simulink model "foc_sensorless_am13x"  (R2025b)
settings: Solver=FixedStepAuto  StartTime=0.0  StopTime=10  RelTol=1e-3  EnableMultiTasking=on
PostLoadFcn:
  | foc_sensorless_am13x_data;
values from neighbouring files (symbols this model uses):
  inverter = mcb.getInverterParameters('BoostXL-DRV8305')    [foc_sensorless_am13x_data.m]
  PI_params = mcb.getPIControllerParameters(pmsm, inverter, PU_System, T_pwm, Ts, Ts_speed)    [foc_sensorless_am13x_data.m]
  pmsm = mcb.getPMSMParameters('Teknic2310P')    [foc_sensorless_am13x_data.m]
  PU_System = mcb.getPUSystemParameters(pmsm, inverter)    [foc_sensorless_am13x_data.m]
  RAMP_STEP_SIZE = Id_init_assumed / N_ramp_steps    (= 0.00025)    [foc_sensorless_am13x_data.m]
  Speed_openLoop_RPM = Speed_openLoop_PU*pmsm.N_base    [foc_sensorless_am13x_data.m]
  T_pwm = 1 / PWM_frequency    (= 5e-05)    [foc_sensorless_am13x_data.m]
  Tclosedloop_stepTime = 5    [foc_sensorless_am13x_data.m]
  Ts = T_pwm    (= 5e-05)    [foc_sensorless_am13x_data.m]
  Ts_motor = T_pwm / 2    (= 2.5e-05)    [foc_sensorless_am13x_data.m]
  Ts_speed = 10 * Ts    (= 0.0005)    [foc_sensorless_am13x_data.m]
  Tspeedchange_stepTime = 7    [foc_sensorless_am13x_data.m]
undefined symbols (not defined in the file or in its folder): ADC_0_INST, DL_ADC_clearInterruptStatus, DL_ADC_INT_NUMBER1, DL_MCPWM_disableTBCLK, target
libraries: mcbcontrolslib x11, mcbeeMathTransformLib x5, simulink x5, slpidlib x3, peripheral_library_blocks_am13x x2, mcbhdlcontrolslib x2, mcbsensorlessestimatorlib x2, mcbpositiondecoderlib x2, mcbplantlib x1, autolibpmsmexterior x1, simulink_extras x1
(part 2 of 2)

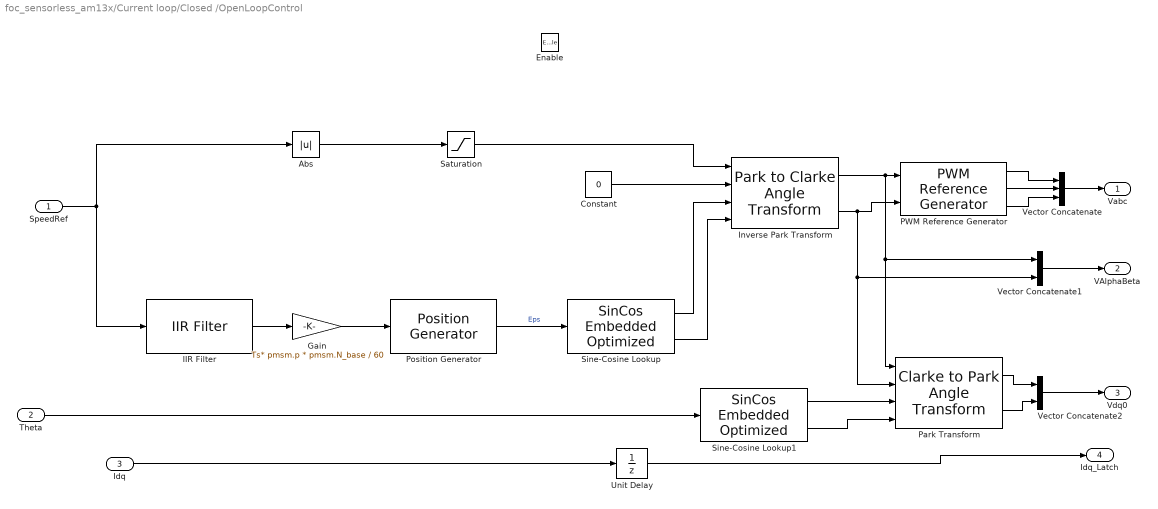
== system foc_sensorless_am13x/Current loop/Closed /OpenLoopControl ==
  SpeedRef : Inport
  Theta : Inport  Port=2
  Idq : Inport  Port=3
  Enable : EnablePort  StatesWhenEnabling=reset
  Abs : Abs  SaturateOnIntegerOverflow=off
  Constant : Constant  Value=0  OutDataTypeStr=dataType
  Gain : Gain  Gain=Ts* pmsm.p * pmsm.N_base / 60  RndMeth=Simplest  OutDataTypeStr=Inherit: Same as input
  IIR Filter : mcbhdlcontrolslib/IIR Filter  VariantControl=Low Pass Filter  VariantSelect=Low-pass  FilterConstantInputType=Specify via dialog  Filter_constant=0.01  advancedSettings=off  Ts=50e-6  cutOff_freq=32.1525
  Inverse Park Transform : mcbeeMathTransformLib/Park to Clarke Angle Transform  AxisAlignment=D-axis  UseWithEmbedded=on  PhaseInput=Two inputs  ThetaInput=Sine and Cosine electrical position  AngleInput=Per-unit  N_points=1024
      settings: LibrarySourceBlock=mcbhdllib/Controls/Math Transforms/Inverse Park Transform
  PWM Reference Generator : mcbcontrolslib/PWM Reference Generator  inSignal=Valphabeta  modType=SVM: space vector modulation
      settings: LibrarySourceBlock=mcblib/Controls/Math Transforms/PWM Reference Generator
  Park Transform : mcbeeMathTransformLib/Clarke to Park Angle Transform  AxisAlignment=D-axis  UseWithEmbedded=on  PhaseInput=Two inputs  ThetaInput=Sine and Cosine electrical position  AngleInput=Per-unit  N_points=1024
      settings: LibrarySourceBlock=mcbhdllib/Controls/Math Transforms/Park Transform
  Position Generator : mcbhdlcontrolslib/Position Generator  AngleOutput=Per-unit  ExternalReset=none  Offset=0
  Saturation : Saturate  LowerLimit=pmsm.V_boost  RndMeth=Simplest
  Sine-Cosine Lookup : mcbcontrolslib/SinCos Embedded Optimized  LabelModeActiveChoice=MCB_Sin  OptforProc=off  ApproximationMethod=None  UserApproxMethod=Lookup  ApproxStatus=None  InterpMethod=Linear point-slope  NumberOfDataPoints=16  NumberOfIterations=11  RemoveProtectionAgainstOutOfRangeInput=off  TableDataTypeStr=Inherit: Inherit via input  AngleInput=Per-unit  ThetaDataType=single  N_points=1024  DatatypeInput=Inherit from input  Datatype=Inherit: Same as input
      settings: LibrarySourceBlock=mcblib/Controls/Math Transforms/Sine-Cosine Lookup
  Sine-Cosine Lookup1 : mcbcontrolslib/SinCos Embedded Optimized  LabelModeActiveChoice=MCB_Sin  OptforProc=off  ApproximationMethod=None  UserApproxMethod=Lookup  ApproxStatus=None  InterpMethod=Linear point-slope  NumberOfDataPoints=16  NumberOfIterations=11  RemoveProtectionAgainstOutOfRangeInput=off  TableDataTypeStr=Inherit: Inherit via input  AngleInput=Per-unit  ThetaDataType=single  N_points=1024  DatatypeInput=Inherit from input  Datatype=Inherit: Same as input
      settings: LibrarySourceBlock=mcblib/Controls/Math Transforms/Sine-Cosine Lookup
  Unit Delay : UnitDelay  SampleTime=-1  HasFrameUpgradeWarning=on
  Vector Concatenate : Concatenate  NumInputs=3
  Vector Concatenate1 : Concatenate
  Vector Concatenate2 : Concatenate
  Vabc : Outport
  VAlphaBeta : Outport  Port=2
  Vdq0 : Outport  Port=3
  Idq_Latch : Outport  Port=4
  wires:
  SpeedRef/1 -> IIR Filter/1, Abs/1
  Abs/1 -> Saturation/1
  Constant/1 -> Inverse Park Transform/2
  IIR Filter/1 -> Gain/1
  Gain/1 -> Position Generator/1
  Position Generator/1 -> Sine-Cosine Lookup/1  "Eps"
  Sine-Cosine Lookup/1 -> Inverse Park Transform/3
  Sine-Cosine Lookup/2 -> Inverse Park Transform/4
  Inverse Park Transform/1 -> Park Transform/1, Vector Concatenate1/1, PWM Reference Generator/1
  Inverse Park Transform/2 -> Park Transform/2, Vector Concatenate1/2, PWM Reference Generator/2
  PWM Reference Generator/3 -> Vector Concatenate/3
  PWM Reference Generator/2 -> Vector Concatenate/2
  PWM Reference Generator/1 -> Vector Concatenate/1
  Vector Concatenate/1 -> Vabc/1
  Vector Concatenate1/1 -> VAlphaBeta/1
  Park Transform/1 -> Vector Concatenate2/1
  Park Transform/2 -> Vector Concatenate2/2
  Vector Concatenate2/1 -> Vdq0/1
  Sine-Cosine Lookup1/1 -> Park Transform/3
  Sine-Cosine Lookup1/2 -> Park Transform/4
  Theta/1 -> Sine-Cosine Lookup1/1
  Saturation/1 -> Inverse Park Transform/1
  Idq/1 -> Unit Delay/1
  Unit Delay/1 -> Idq_Latch/1

== system foc_sensorless_am13x/Current loop/Closed /OutputScaling ==
  VabcClosed : Inport
  VabcOpen : Inport  Port=2
  EnCl : Inport  Port=3  OutDataTypeStr=boolean
  Mode : Inport  Port=4
  Add2 : Sum
  Constant : Constant  Value=0.5  OutDataTypeStr=dataType
  Current Offset Calib : Constant  Value=[0.5 0.5 0.5]  OutDataTypeStr=dataType
  Gain : Gain  Gain=0.5  RndMeth=Simplest  OutDataTypeStr=Inherit: Same as input
  Switch : Switch  Criteria=u2 > Threshold  SaturateOnIntegerOverflow=off  InputSameDT=off
  Switch3 : Switch  Criteria=u2 > Threshold  SaturateOnIntegerOverflow=off  InputSameDT=off
  Vabc_PU : Outport  OutDataTypeStr=single  VectorParamsAs1DForOutWhenUnconnected=off
  wires:
  VabcClosed/1 -> Switch/1
  EnCl/1 -> Switch/2
  Gain/1 -> Add2/1
  VabcOpen/1 -> Switch/3
  Constant/1 -> Add2/2
  Switch/1 -> Gain/1
  Switch3/1 -> Vabc_PU/1
  Mode/1 -> Switch3/2
  Add2/1 -> Switch3/1
  Current Offset Calib/1 -> Switch3/3

== system foc_sensorless_am13x/Current loop/Closed /Sensorless algorithms to calculate position and speed ==
  note: Try different sensorless algorithms
  EnPWM : Inport
  VI_fb : Inport  Port=2
  Data Store Memory : DataStoreMemory  DataStoreName=Enable  WriteAfterWriteMsg=warning  ShowAdditionalParam=off
  Data Store Write : DataStoreWrite  DataStoreName=Enable  DataStoreElements=Enable  IndexOptions=Index vector (dialog)  Indices=1  OutputSizes=1
  Demux : Demux  Outputs=2
  EstimatorSelector : Constant  Value=2  OutDataTypeStr=uint32
  Extended EMF Observer : Subsystem
  Flux Observer : Subsystem
  Merge : Merge  Inputs=3
  Sliding Mode Observer : Subsystem
  Switch Case : SwitchCase  CaseConditions={0,1,2}  ShowDefaultCase=off
  Pos_PU : Outport
  speed_PU : Outport  Port=2
  wires:
  Switch Case/3 -> Extended EMF Observer/Action
  Extended EMF Observer/1(Position/Speed) -> Merge/3
  VI_fb/1 -> Sliding Mode Observer/1(InputSignals), Flux Observer/1(InputSignals), Extended EMF Observer/1(InputSignals)
  Switch Case/1 -> Sliding Mode Observer/Action
  Switch Case/2 -> Flux Observer/Action
  Merge/1 -> Demux/1
  Flux Observer/1(Position/Speed) -> Merge/2
  Sliding Mode Observer/1(Position/Speed) -> Merge/1
  EstimatorSelector/1 -> Switch Case/1
  Demux/2 -> speed_PU/1
  Demux/1 -> Pos_PU/1
  EnPWM/1 -> Data Store Write/1

== system foc_sensorless_am13x/Current loop/Create Buffer/Data ==
  Data : Inport
  Data_width : Inport  Port=2
  Action Port : ActionPort  ActionPortLabel=else
  Mux : Mux  Inputs=2
  Start : Constant  Value=hex2dec('0000')  OutDataTypeStr=uint16
  Data_out : Outport  VectorParamsAs1DForOutWhenUnconnected=off
  Iteration : Outport  Port=2  VectorParamsAs1DForOutWhenUnconnected=off
  wires:
  Start/1 -> Mux/2
  Mux/1 -> Data_out/1
  Data/1 -> Mux/1
  Data_width/1 -> Iteration/1

== system foc_sensorless_am13x/Current loop/Create Buffer/Data_Conditioning ==
  In1 : Inport
  Data Type Conversion : DataTypeConversion  OutDataTypeStr=fixdt(1,32,12)  RndMeth=Simplest  SaturateOnIntegerOverflow=off
  Data Type Conversion3 : DataTypeConversion  OutDataTypeStr=uint16  ConvertRealWorld=Stored Integer (SI)  RndMeth=Simplest  SaturateOnIntegerOverflow=off
  Out1 : Outport  VectorParamsAs1DForOutWhenUnconnected=off
  wires:
  In1/1 -> Data Type Conversion/1
  Data Type Conversion3/1 -> Out1/1
  Data Type Conversion/1 -> Data Type Conversion3/1

== system foc_sensorless_am13x/Current loop/Create Buffer/End ==
  Data : Inport
  Data_width : Inport  Port=2
  Action Port : ActionPort  ActionPortLabel=elseif(u1 == 599)
  Bias : Bias  Bias=1  SaturateOnIntegerOverflow=off
  Mux : Mux  Inputs=2
  Start : Constant  Value=hex2dec('4545')  OutDataTypeStr=uint16
  Data_out : Outport  VectorParamsAs1DForOutWhenUnconnected=off
  Iteration : Outport  Port=2  VectorParamsAs1DForOutWhenUnconnected=off
  wires:
  Mux/1 -> Data_out/1
  Data_width/1 -> Bias/1
  Start/1 -> Mux/2
  Bias/1 -> Iteration/1
  Data/1 -> Mux/1

== system foc_sensorless_am13x/Current loop/Create Buffer/Start ==
  Data : Inport
  Data_width : Inport  Port=2
  Action Port : ActionPort  ActionPortLabel=if(u1 == 0)
  Bias : Bias  Bias=1  SaturateOnIntegerOverflow=off
  End : Constant  Value=hex2dec('5353')  OutDataTypeStr=uint16
  Mux : Mux  Inputs=2
  Data_out : Outport  VectorParamsAs1DForOutWhenUnconnected=off
  Iteration : Outport  Port=2  VectorParamsAs1DForOutWhenUnconnected=off
  wires:
  End/1 -> Mux/1
  Mux/1 -> Data_out/1
  Data_width/1 -> Bias/1
  Bias/1 -> Iteration/1
  Data/1 -> Mux/2

== system foc_sensorless_am13x/Current loop/Serial Send/While Iterator Subsystem ==
  note: UART configuration is done via HAL APIs
      | - Its hardcoded for 5e6 baud refer the source am13x_serial_util.c
  Data : Inport
  Iteration : Inport  Port=2
  Add : Sum  Inputs=+-  OutDataTypeStr=Inherit: Same as first input
  HAL Serial API Caller : CFunction  CodeGenUsesSimCustomCode=off  CodegenOutputCode=mw_am13x_serial_Send((const uint8_t *)&serialIn, sizeof(uint16_t));  CustomHeaderFile=|  CustomSourceFile=am13x_serial_util.c
      | dl_mcpwm.h
      | hw_memmap.h
      | ti_sdk_dl_config.h
      | Uart_Hal.h
      | dl_gpio.h
      | mw_am13x_serial.h
  Index Vector : MultiPortSwitch  Inputs=1  SaturateOnIntegerOverflow=off  InputSameDT=off
  While Iterator : WhileIterator  MaxIters=-1  WhileBlockType=do-while  ShowIterationPort=on  OutputDataType=int16
  wires:
  While Iterator/1 -> Add/2, Index Vector/1
  Data/1 -> Index Vector/2
  Add/1 -> While Iterator/1
  Iteration/1 -> Add/1
  Index Vector/1 -> HAL Serial API Caller/1

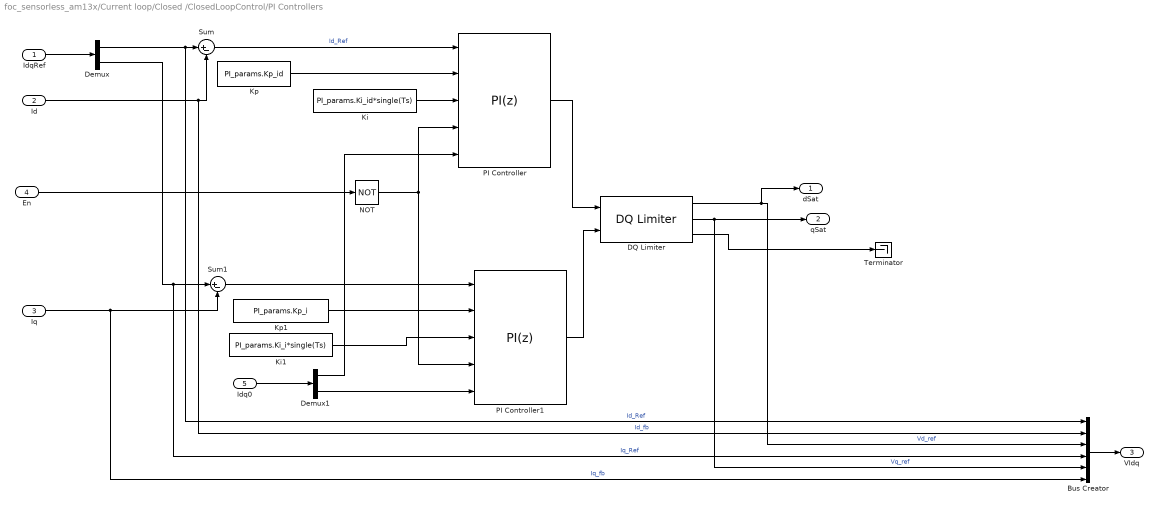
== system foc_sensorless_am13x/Current loop/Closed /ClosedLoopControl/PI Controllers ==
  IdqRef : Inport
  Id : Inport  Port=2
  Iq : Inport  Port=3
  En : Inport  Port=4
  Idq0 : Inport  Port=5
  Bus Creator : BusCreator  Inputs=6
  DQ Limiter : mcbcontrolslib/DQ Limiter  satMethodInputType=Specify via dialog  satMethodSelected=D-Q equivalence  satLimitInputType=Specify via dialog  Vmax=.95
      settings: LibrarySourceBlock=mcblib/Controls/Control Reference/DQ Limiter
  Demux : Demux  Outputs=2
  Demux1 : Demux  Outputs=2
  Ki : Constant  Value=PI_params.Ki_id*single(Ts)  OutDataTypeStr=dataType  SampleTime=-1
  Ki1 : Constant  Value=PI_params.Ki_i*single(Ts)  OutDataTypeStr=dataType  SampleTime=-1
  Kp : Constant  Value=PI_params.Kp_id  OutDataTypeStr=dataType  SampleTime=-1
  Kp1 : Constant  Value=PI_params.Kp_i  OutDataTypeStr=dataType  SampleTime=-1
  NOT : Logic  Operator=NOT  IconShape=distinctive  AllPortsSameDT=off  OutDataTypeStr=boolean
  PI Controller : slpidlib/PID Controller  Controller=PI  Form=Parallel  TimeDomain=Discrete-time  UseExternalTs=off  SampleTime=-1  IntegratorMethod=Forward Euler  FilterMethod=Forward Euler  ControllerParametersSource=external  P=1  I=1  UseKiTs=on  D=0  UseExternalDerivativeSource=off  N=100  UseFilter=on  TunerSelectOption=Transfer Function Based (PID Tuner App)  InitialConditionSource=external  InitialConditionForIntegrator=0  InitialConditionForFilter=0  DifferentiatorICPrevScaledInput=0  ExternalReset=level  TrackingMode=off  Kt=1  LimitOutput=on  SatLimitsSource=internal  UpperSaturationLimit=1  LowerSaturationLimit=-1  LinearizeAsGain=on  AntiWindupMode=clamping  Kb=1  LimitIntegrator=off  UpperIntegratorSaturationLimit=inf  LowerIntegratorSaturationLimit=-inf  RndMeth=Simplest  POutMin=[]  POutMax=[]  IOutMin=[]  IOutMax=[]  DOutMin=[]  DOutMax=[]  NOutMin=[]  NOutMax=[]  SumOutMin=[]  SumOutMax=[]  SaturationOutDataTypeStr=Inherit: Inherit via back propagation  SaturationOutMin=[]  SaturationOutMax=[]  PParamMin=[]  PParamMax=[]  IParamMin=[]  IParamMax=[]  DParamMin=[]  DParamMax=[]  NParamMin=[]  NParamMax=[]  KbParamMin=[]  KbParamMax=[]  KtParamMin=[]  KtParamMax=[]  KbOutMin=[]  KbOutMax=[]  KtOutMin=[]  KtOutMax=[]  IntegratorOutMin=[]  IntegratorOutMax=[]  FilterOutMin=[]  FilterOutMax=[]  SumI1OutMin=[]  SumI1OutMax=[]  SumI2OutMin=[]  SumI2OutMax=[]  SumI3OutMin=[]  SumI3OutMax=[]  SumI4OutMin=[]  SumI4OutMax=[]  SumDOutMin=[]  SumDOutMax=[]  DifferentiatorOutMin=[]  DifferentiatorOutMax=[]  FilterDiffOutCoefMin=[]  FilterDiffOutCoefMax=[]  ReciprocalOutMin=[]  ReciprocalOutMax=[]  SumDenOutMin=[]  SumDenOutMax=[]  SumNumOutMin=[]  SumNumOutMax=[]  DivideOutMin=[]  DivideOutMax=[]  UdiffTsProdOutMin=[]  UdiffTsProdOutMax=[]  NTsProdOutMin=[]  NTsProdOutMax=[]  UintegralTsProdOutMin=[]  UintegralTsProdOutMax=[]  UngainTsProdOutMin=[]  UngainTsProdOutMax=[]  ClampingZeroOutDataTypeStr=Inherit: Inherit via back propagation  ClampingZeroOutMin=[]  ClampingZeroOutMax=[]  FilterDenConstantOutDataTypeStr=Inherit: Inherit via back propagation  FilterDenConstantOutMin=[]  FilterDenConstantOutMax=[]  PCopyOutDataTypeStr=Inherit: Inherit via back propagation  PCopyOutMin=[]  PCopyOutMax=[]  NCopyOutDataTypeStr=Inherit: Inherit via back propagation  NCopyOutMin=[]  NCopyOutMax=[]  IntegratorContinuousStateAttributes=''  IntegratorStateMustResolveToSignalObject=off  IntegratorRTWStateStorageClass=Auto  FilterContinuousStateAttributes=''  FilterStateMustResolveToSignalObject=off  FilterRTWStateStorageClass=Auto  ParallelPVariant=ExternalParameters  IdealPVariant=Disabled  IVariant=ExternalParameters  DVariant=Disabled  IntegratorVariant=Discrete  SatVariant=Enabled  AWVariant=DiscClampingParallel  PCopyVariant=Disabled  TRVariant=Disabled  FdbkBlocksVariant=Forward  IdealPFdbkVariant=Disabled  SatFdbkVariant=Disabled  DerivativeFilterVariant=Disabled  NVariant=Disabled  NCopyVariant=Disabled_SignalSpec  FilterICVariant=Disabled  IntegratorICVariant=ExternalICs  ExternalResetVariant=ExternalReset  TRSumVariant=Passthrough  SumFdbkVariant=Disabled  SumVariant=Sum_PI  TsampFilterVariant=InternalTs  TsampNgainVariant=Passthrough  TsampIntegralVariant=Disabled_SignalSpec  ExternalSaturationOutDataTypeStr=Inherit: Same as second input  DerivativeSourceVariant=Disabled  PreIntVariant=InternalPreInt
      settings: LibrarySourceBlock=mcblib/Controls/Controllers/PI Controller
  PI Controller1 : slpidlib/PID Controller  Controller=PI  Form=Parallel  TimeDomain=Discrete-time  UseExternalTs=off  SampleTime=-1  IntegratorMethod=Forward Euler  FilterMethod=Forward Euler  ControllerParametersSource=external  P=1  I=1  UseKiTs=on  D=0  UseExternalDerivativeSource=off  N=100  UseFilter=on  TunerSelectOption=Transfer Function Based (PID Tuner App)  InitialConditionSource=external  InitialConditionForIntegrator=0  InitialConditionForFilter=0  DifferentiatorICPrevScaledInput=0  ExternalReset=level  TrackingMode=off  Kt=1  LimitOutput=on  SatLimitsSource=internal  UpperSaturationLimit=1  LowerSaturationLimit=-1  LinearizeAsGain=on  AntiWindupMode=clamping  Kb=1  LimitIntegrator=off  UpperIntegratorSaturationLimit=inf  LowerIntegratorSaturationLimit=-inf  RndMeth=Simplest  POutMin=[]  POutMax=[]  IOutMin=[]  IOutMax=[]  DOutMin=[]  DOutMax=[]  NOutMin=[]  NOutMax=[]  SumOutMin=[]  SumOutMax=[]  SaturationOutDataTypeStr=Inherit: Inherit via back propagation  SaturationOutMin=[]  SaturationOutMax=[]  PParamMin=[]  PParamMax=[]  IParamMin=[]  IParamMax=[]  DParamMin=[]  DParamMax=[]  NParamMin=[]  NParamMax=[]  KbParamMin=[]  KbParamMax=[]  KtParamMin=[]  KtParamMax=[]  KbOutMin=[]  KbOutMax=[]  KtOutMin=[]  KtOutMax=[]  IntegratorOutMin=[]  IntegratorOutMax=[]  FilterOutMin=[]  FilterOutMax=[]  SumI1OutMin=[]  SumI1OutMax=[]  SumI2OutMin=[]  SumI2OutMax=[]  SumI3OutMin=[]  SumI3OutMax=[]  SumI4OutMin=[]  SumI4OutMax=[]  SumDOutMin=[]  SumDOutMax=[]  DifferentiatorOutMin=[]  DifferentiatorOutMax=[]  FilterDiffOutCoefMin=[]  FilterDiffOutCoefMax=[]  ReciprocalOutMin=[]  ReciprocalOutMax=[]  SumDenOutMin=[]  SumDenOutMax=[]  SumNumOutMin=[]  SumNumOutMax=[]  DivideOutMin=[]  DivideOutMax=[]  UdiffTsProdOutMin=[]  UdiffTsProdOutMax=[]  NTsProdOutMin=[]  NTsProdOutMax=[]  UintegralTsProdOutMin=[]  UintegralTsProdOutMax=[]  UngainTsProdOutMin=[]  UngainTsProdOutMax=[]  ClampingZeroOutDataTypeStr=Inherit: Inherit via back propagation  ClampingZeroOutMin=[]  ClampingZeroOutMax=[]  FilterDenConstantOutDataTypeStr=Inherit: Inherit via back propagation  FilterDenConstantOutMin=[]  FilterDenConstantOutMax=[]  PCopyOutDataTypeStr=Inherit: Inherit via back propagation  PCopyOutMin=[]  PCopyOutMax=[]  NCopyOutDataTypeStr=Inherit: Inherit via back propagation  NCopyOutMin=[]  NCopyOutMax=[]  IntegratorContinuousStateAttributes=''  IntegratorStateMustResolveToSignalObject=off  IntegratorRTWStateStorageClass=Auto  FilterContinuousStateAttributes=''  FilterStateMustResolveToSignalObject=off  FilterRTWStateStorageClass=Auto  ParallelPVariant=ExternalParameters  IdealPVariant=Disabled  IVariant=ExternalParameters  DVariant=Disabled  IntegratorVariant=Discrete  SatVariant=Enabled  AWVariant=DiscClampingParallel  PCopyVariant=Disabled  TRVariant=Disabled  FdbkBlocksVariant=Forward  IdealPFdbkVariant=Disabled  SatFdbkVariant=Disabled  DerivativeFilterVariant=Disabled  NVariant=Disabled  NCopyVariant=Disabled_SignalSpec  FilterICVariant=Disabled  IntegratorICVariant=ExternalICs  ExternalResetVariant=ExternalReset  TRSumVariant=Passthrough  SumFdbkVariant=Disabled  SumVariant=Sum_PI  TsampFilterVariant=InternalTs  TsampNgainVariant=Passthrough  TsampIntegralVariant=Disabled_SignalSpec  ExternalSaturationOutDataTypeStr=Inherit: Same as second input  DerivativeSourceVariant=Disabled  PreIntVariant=InternalPreInt
      settings: LibrarySourceBlock=mcblib/Controls/Controllers/PI Controller
  Sum : Sum  Inputs=|+-
  Sum1 : Sum  Inputs=|+-
  Terminator : Terminator
  dSat : Outport
  qSat : Outport  Port=2
  VIdq : Outport  Port=3  VectorParamsAs1DForOutWhenUnconnected=off
  wires:
  DQ Limiter/3 -> Terminator/1
  PI Controller/1 -> DQ Limiter/1
  Sum1/1 -> PI Controller1/1
  DQ Limiter/1 -> Bus Creator/3, dSat/1  "Vd_ref"
  PI Controller1/1 -> DQ Limiter/2
  IdqRef/1 -> Demux/1
  Demux/1 -> Bus Creator/1, Sum/1  "Id_Ref"
  Kp/1 -> PI Controller/2
  Ki/1 -> PI Controller/3
  Kp1/1 -> PI Controller1/2
  Ki1/1 -> PI Controller1/3
  En/1 -> NOT/1
  NOT/1 -> PI Controller/4, PI Controller1/4
  Idq0/1 -> Demux1/1
  Id/1 -> Bus Creator/2, Sum/2  "Id_fb"
  Sum/1 -> PI Controller/1  "Id_Ref"
  Bus Creator/1 -> VIdq/1
  DQ Limiter/2 -> Bus Creator/5, qSat/1  "Vq_ref"
  Iq/1 -> Bus Creator/6, Sum1/2  "Iq_fb"
  Demux/2 -> Bus Creator/4, Sum1/1  "Iq_Ref"
  Demux1/1 -> PI Controller/5
  Demux1/2 -> PI Controller1/5

== system foc_sensorless_am13x/Current loop/Closed /Compensate ADC offset/Enabled Subsystem ==
  Iab_ADC : Inport
  Enable : EnablePort
  Add : Sum
  Add1 : Sum
  Constant : Constant  OutDataTypeStr=uint32  SampleTime=-1
  Divide : Product  Inputs=*/
  Gain : Gain  Gain=1e-3  OutDataTypeStr=dataType  RndMeth=Simplest
  Gain1 : Gain  Gain=1e3  OutDataTypeStr=uint16
  Unit Delay : UnitDelay  SampleTime=-1  HasFrameUpgradeWarning=on
  Unit Delay1 : UnitDelay  SampleTime=-1  HasFrameUpgradeWarning=on
  Iab_Offset : Outport  InitialOutput=2048
  wires:
  Gain1/1 -> Iab_Offset/1
  Divide/1 -> Gain1/1
  Add1/1 -> Unit Delay1/1, Divide/2
  Unit Delay1/1 -> Add1/2
  Constant/1 -> Add1/1
  Add/1 -> Unit Delay/1, Divide/1
  Unit Delay/1 -> Add/2
  Gain/1 -> Add/1
  Iab_ADC/1 -> Gain/1

== system foc_sensorless_am13x/Current loop/Closed /Sensorless algorithms to calculate position and speed/Extended EMF Observer ==
  InputSignals : Inport
  Action Port : ActionPort  ActionPortLabel=case [ 2 ]:
  Data Store Read1 : DataStoreRead  DataStoreName=Enable  IndexOptions=Index vector (dialog)  Indices=1  OutputSizes=1
  Demux1 : Demux
  Extended EMF Observer : mcbsensorlessestimatorlib/Extended EMF Observer  ParameterBusInput=off  InputUnit=Per-unit  PosOut=Electrical position  BlkSampleTime=Ts  StatorResistance=pmsm.Rs  StatorDaxisInductance=pmsm.Ld  StatorQaxisInductance=pmsm.Lq  MaxApplicationSpeed=pmsm.N_base  PolePairs=pmsm.p  MaxStatorVoltage=PU_System.V_base  MaxStatorCurrent=PU_System.I_base  Alpha=10  EEMFCutoffFreq=7500  Kp=250  Ki=200000  N_points=1024  SpeedCutoffFreq=15  PositionUnit=Per-unit  PositionDataType=dataType  SpeedUnit=Per-unit  PerUnitSpeed=PU_System.N_base  SpeedDataType=dataType  TableDatatype=single
      settings: LibrarySourceBlock=mcblib/Sensorless Estimators/Extended EMF Observer
  Logical Operator : Logic  Operator=NOT  IconShape=distinctive  AllPortsSameDT=off  OutDataTypeStr=boolean
  Mux2 : Mux  Inputs=2
  Position/Speed : Outport
  wires:
  Extended EMF Observer/2 -> Mux2/2
  Extended EMF Observer/1 -> Mux2/1
  InputSignals/1 -> Demux1/1
  Demux1/2 -> Extended EMF Observer/2
  Demux1/1 -> Extended EMF Observer/1
  Data Store Read1/1 -> Logical Operator/1
  Logical Operator/1 -> Extended EMF Observer/5
  Demux1/4 -> Extended EMF Observer/4  "Ibeta"
  Demux1/3 -> Extended EMF Observer/3  "Ialpha"
  Mux2/1 -> Position/Speed/1

== system foc_sensorless_am13x/Current loop/Closed /Sensorless algorithms to calculate position and speed/Flux Observer ==
  note: error xternal Mode Open Protocol Connect command failed Caused by: Error in 'OpenLoop_AM13x_withADC/Open Loop/Monitoring/Calculate position and speed/Flux Observer/Flux Observer': Failed to evaluate mask initialization commands. Cannot change property 'Enabled' of 'OpenLoop_AM13x_withADC/Open Loop/Monitoring/Calculate position and speed/Flux Observer/Flux Observer' while simulation is running Component:Simulink | Category:Model error Unable to connect to the 'AM13E230x' target for 'OpenLoop_AM13x_withADC'. Component:Simulink | Category:Block diagram error
  InputSignals : Inport
  Action Port : ActionPort  ActionPortLabel=case [ 1 ]:
  DC component removal : Subsystem
  DC component removal1 : Subsystem  Commented=through
  Data Store Read1 : DataStoreRead  DataStoreName=Enable  IndexOptions=Index vector (dialog)  Indices=1  OutputSizes=1
  Demux1 : Demux
  Flux Observer : mcbpositiondecoderlib/Flux Observer  DataTypeSelect=off  ParameterBusInput=off  MotorSelection=PMSM  BlockInputUnit=Per-unit  PerUnitVoltage=PU_System.V_base  PerUnitCurrent=PU_System.I_base  PositionSelect=on  FluxSelect=off  TorqueSelect=off  PolePairs=pmsm.p  StatorResistance=pmsm.Rs  StatorDAxisInductance=pmsm.Ld  StatorLeakageInductance=0.0068  RotorLeakageInductance=0.0068  MagnetizingInductance=0.0300  CutoffFreq=3.1863  BlockSampleTime=Ts  PositionUnit=Per-unit  PositionDatatype=dataType  FluxUnit=Weber  PerUnitFlux=0.1  FluxDatatype=single  TorqueUnit=Nm  PerUnitTorque=100  TorqueDatatype=single  DataType=0
  IIR Filter4 : mcbcontrolslib/IIR Filter  VariantControl=Low Pass Filter  VariantSelect=Low-pass  FilterConstantInputType=Specify via dialog  Filter_constant=0.01  InitialOutput=Specify via dialog  InitialOutputValue=0  ExternalReset=none  advancedSettings=on  Ts=50e-6  cutOff_freq=32.1525
  Logical Operator : Logic  Operator=NOT  IconShape=distinctive  AllPortsSameDT=off  OutDataTypeStr=boolean
  Mux2 : Mux  Inputs=2
  Speed Measurement : mcbpositiondecoderlib/Speed Measurement  DiscreteStepInput=off  LastDiscreteStepInput=off  PositionUnit=Per unit  PositionScalingDatatype=uint32  SpeedCalculationMode=Time interval for speed calculation  TempSpeedCalculationMode=Time interval for speed calculation  SampleTimeAsync=Ts  MaximumApplicationSpeed=60000  SpeedResolution=5e-6  DelayLength=10  MaximumMeasurableSpeed=54545.4545  MeasurableSpeedResolution=2.794e-05  SpeedUnit=Per unit based on dialog  TempSpeedUnit=RPM  PerUnitSpeed=PU_System.N_base  SpeedDataType=dataType
  elect2mech : Gain  Gain=1/pmsm.p  RndMeth=Simplest  OutDataTypeStr=Inherit: Same as input
  Position/Speed : Outport
  wires:
  DC component removal/1(SigOUT) -> Demux1/1
  Demux1/2 -> Flux Observer/2
  Demux1/1 -> Flux Observer/1
  Flux Observer/1 -> Speed Measurement/1, Mux2/1
  Data Store Read1/1 -> Logical Operator/1
  Logical Operator/1 -> Flux Observer/5
  IIR Filter4/1 -> elect2mech/1
  Demux1/4 -> Flux Observer/4  "Ibeta"
  Demux1/3 -> Flux Observer/3  "Ialpha"
  elect2mech/1 -> Mux2/2
  Speed Measurement/1 -> IIR Filter4/1
  Mux2/1 -> Position/Speed/1
  InputSignals/1 -> DC component removal/1(SigIN)

== system foc_sensorless_am13x/Current loop/Closed /Sensorless algorithms to calculate position and speed/Sliding Mode Observer ==
  InputSignals : Inport
  Action Port : ActionPort  ActionPortLabel=case [ 0 ]:
  Data Store Read1 : DataStoreRead  DataStoreName=Enable  IndexOptions=Index vector (dialog)  Indices=1  OutputSizes=1
  Demux1 : Demux
  Logical Operator : Logic  Operator=NOT  IconShape=distinctive  AllPortsSameDT=off  OutDataTypeStr=boolean
  Mux : Mux  Inputs=2
  Sliding Mode Observer : mcbsensorlessestimatorlib/Sliding Mode Observer  InputUnit=Per-unit  BlkSampleTime=Ts  StatorResistance=pmsm.Rs  StatorInductance=pmsm.Ld  MaxApplicationSpeed=pmsm.N_base  PolePairs=pmsm.p  MaxStatorVoltage=PU_System.V_base  MaxStatorCurrent=PU_System.I_base  DisturbanceObserverGain=smo.BackEmfObsGain  CurrentObserverGain=smo.CurrentObsGain  CutoffFreq=smo.CutoffFreq  PositionUnit=Per unit  PositionDataType=dataType  SpeedUnit=Per unit  PerUnitSpeed=PU_System.N_base  SpeedDataType=dataType
  Position/Speed : Outport
  wires:
  Demux1/2 -> Sliding Mode Observer/2
  Demux1/1 -> Sliding Mode Observer/1
  Sliding Mode Observer/2 -> Mux/2
  Logical Operator/1 -> Sliding Mode Observer/5
  Data Store Read1/1 -> Logical Operator/1
  InputSignals/1 -> Demux1/1
  Sliding Mode Observer/1 -> Mux/1
  Demux1/3 -> Sliding Mode Observer/3  "Ialpha"
  Demux1/4 -> Sliding Mode Observer/4  "Ibeta"
  Mux/1 -> Position/Speed/1

== system foc_sensorless_am13x/Current loop/Closed /Sensorless algorithms to calculate position and speed/Flux Observer/DC component removal ==
  SigIN : Inport
  IIR Filter : mcbcontrolslib/IIR Filter  VariantControl=Low Pass Filter  VariantSelect=High-pass  FilterConstantInputType=Specify via dialog  Filter_constant=0.0005*(Ts/50e-6)  InitialOutput=Specify via dialog  InitialOutputValue=0  ExternalReset=none  advancedSettings=on  Ts=50e-6  cutOff_freq=1.5923
  SigOUT : Outport
  wires:
  IIR Filter/1 -> SigOUT/1
  SigIN/1 -> IIR Filter/1

== system foc_sensorless_am13x/Current loop/Closed /Sensorless algorithms to calculate position and speed/Flux Observer/DC component removal1 ==
  SigIN : Inport
  IIR Filter : mcbcontrolslib/IIR Filter  VariantControl=Low Pass Filter  VariantSelect=Low-pass  FilterConstantInputType=Specify via dialog  Filter_constant=0.005*(Ts/50e-6)  InitialOutput=Specify via dialog  InitialOutputValue=0  ExternalReset=none  advancedSettings=on  Ts=50e-6  cutOff_freq=1
  Sum6 : Sum  Inputs=|+-  RndMeth=Simplest  OutDataTypeStr=Inherit: Same as first input
  SigOUT : Outport
  wires:
  IIR Filter/1 -> Sum6/2
  SigIN/1 -> IIR Filter/1, Sum6/1
  Sum6/1 -> SigOUT/1
